simulink model "TST_EngPrt_PrtLimMech"  (R2016b)
settings: Solver=FixedStepDiscrete  StartTime=0.0  StopTime=simTime  FixedStep=sampleTime  RelTol=1e-3
values from neighbouring files (symbols this model uses):
  testCase = 1    [initTST_EngPrt_PrtLimMech_001.m]    (also in initTST_EngPrt_PrtLimMech_002.m = 2; initTST_EngPrt_PrtLimMech_003.m = 3; initTST_EngPrt_PrtLimMech_004.m = 4)
libraries: simulink x17, UnitTest_Lib x12
settings Model: Creator=zhengjinyan  LastModifiedBy=zhengjinyan
settings DebuggingCC: SignalRangeChecking=error

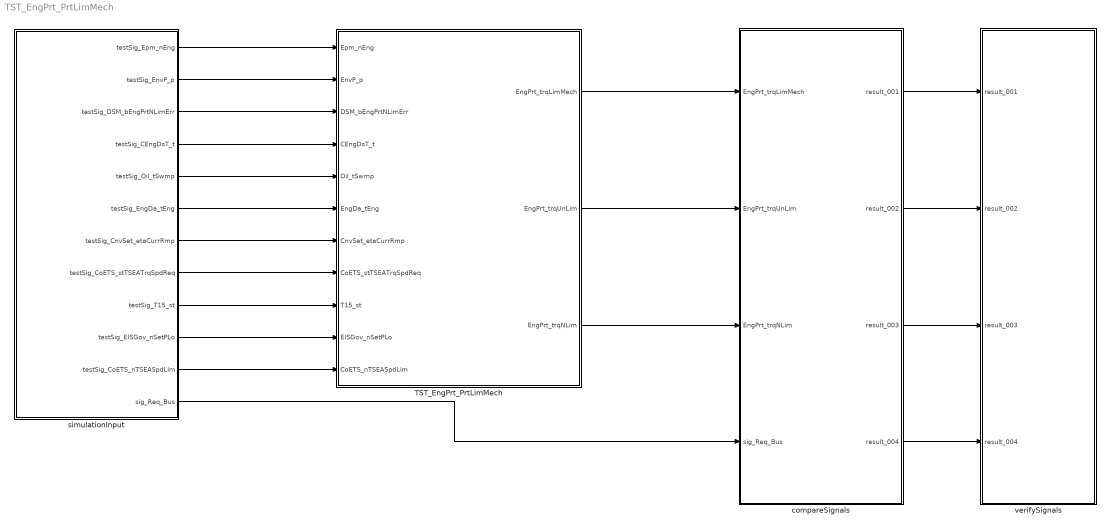
== system TST_EngPrt_PrtLimMech ==
  TST_EngPrt_PrtLimMech : Subsystem
  compareSignals : Subsystem
  simulationInput : Subsystem
  verifySignals : Subsystem
  wires:
  simulationInput/1(testSig_Epm_nEng) -> TST_EngPrt_PrtLimMech/1(Epm_nEng)
  simulationInput/2(testSig_EnvP_p) -> TST_EngPrt_PrtLimMech/2(EnvP_p)
  simulationInput/3(testSig_DSM_bEngPrtNLimErr) -> TST_EngPrt_PrtLimMech/3(DSM_bEngPrtNLimErr)
  simulationInput/4(testSig_CEngDsT_t) -> TST_EngPrt_PrtLimMech/4(CEngDsT_t)
  simulationInput/5(testSig_Oil_tSwmp) -> TST_EngPrt_PrtLimMech/5(Oil_tSwmp)
  simulationInput/6(testSig_EngDa_tEng) -> TST_EngPrt_PrtLimMech/6(EngDa_tEng)
  simulationInput/7(testSig_CnvSet_etaCurrRmp) -> TST_EngPrt_PrtLimMech/7(CnvSet_etaCurrRmp)
  simulationInput/8(testSig_CoETS_stTSEATrqSpdReq) -> TST_EngPrt_PrtLimMech/8(CoETS_stTSEATrqSpdReq)
  simulationInput/9(testSig_T15_st) -> TST_EngPrt_PrtLimMech/9(T15_st)
  simulationInput/10(testSig_EISGov_nSetPLo) -> TST_EngPrt_PrtLimMech/10(EISGov_nSetPLo)
  simulationInput/11(testSig_CoETS_nTSEASpdLim) -> TST_EngPrt_PrtLimMech/11(CoETS_nTSEASpdLim)
  TST_EngPrt_PrtLimMech/1(EngPrt_trqLimMech) -> compareSignals/1(EngPrt_trqLimMech)
  TST_EngPrt_PrtLimMech/2(EngPrt_trqUnLim) -> compareSignals/2(EngPrt_trqUnLim)
  TST_EngPrt_PrtLimMech/3(EngPrt_trqNLim) -> compareSignals/3(EngPrt_trqNLim)
  simulationInput/12(sig_Req_Bus) -> compareSignals/4(sig_Req_Bus)
  compareSignals/1(result_001) -> verifySignals/1(result_001)
  compareSignals/2(result_002) -> verifySignals/2(result_002)
  compareSignals/3(result_003) -> verifySignals/3(result_003)
  compareSignals/4(result_004) -> verifySignals/4(result_004)

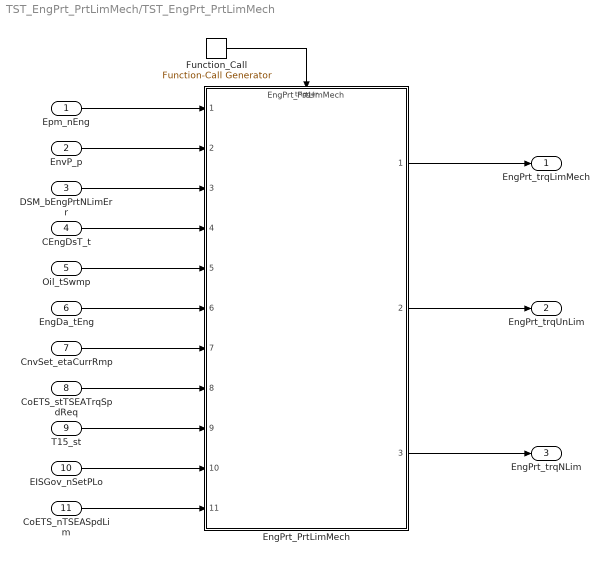
== system TST_EngPrt_PrtLimMech/TST_EngPrt_PrtLimMech ==
  Epm_nEng : Inport
  EnvP_p : Inport  Port=2
  DSM_bEngPrtNLimErr : Inport  Port=3
  CEngDsT_t : Inport  Port=4
  Oil_tSwmp : Inport  Port=5
  EngDa_tEng : Inport  Port=6
  CnvSet_etaCurrRmp : Inport  Port=7
  CoETS_stTSEATrqSpdReq : Inport  Port=8
  T15_st : Inport  Port=9
  EISGov_nSetPLo : Inport  Port=10
  CoETS_nTSEASpdLim : Inport  Port=11
  EngPrt_PrtLimMech : ModelReference  ModelNameDialog=EngPrt_PrtLimMech  SimulationMode=Normal  ModelReferenceVersion=1.43  TriggerPortName=function  TriggerPortTriggerType=function-call  TriggerPortStatesWhenEnabling=held
  Function_Call : simulink/Ports & Subsystems/Function-Call Generator  sample_time=sampleTime  numberOfIterations=1
  EngPrt_trqLimMech : Outport
  EngPrt_trqUnLim : Outport  Port=2
  EngPrt_trqNLim : Outport  Port=3
  wires:
  Function_Call/1 -> EngPrt_PrtLimMech/Trigger
  Epm_nEng/1 -> EngPrt_PrtLimMech/1
  EnvP_p/1 -> EngPrt_PrtLimMech/2
  DSM_bEngPrtNLimErr/1 -> EngPrt_PrtLimMech/3
  CEngDsT_t/1 -> EngPrt_PrtLimMech/4
  Oil_tSwmp/1 -> EngPrt_PrtLimMech/5
  EngDa_tEng/1 -> EngPrt_PrtLimMech/6
  CnvSet_etaCurrRmp/1 -> EngPrt_PrtLimMech/7
  CoETS_stTSEATrqSpdReq/1 -> EngPrt_PrtLimMech/8
  T15_st/1 -> EngPrt_PrtLimMech/9
  EISGov_nSetPLo/1 -> EngPrt_PrtLimMech/10
  CoETS_nTSEASpdLim/1 -> EngPrt_PrtLimMech/11
  EngPrt_PrtLimMech/1 -> EngPrt_trqLimMech/1
  EngPrt_PrtLimMech/2 -> EngPrt_trqUnLim/1
  EngPrt_PrtLimMech/3 -> EngPrt_trqNLim/1

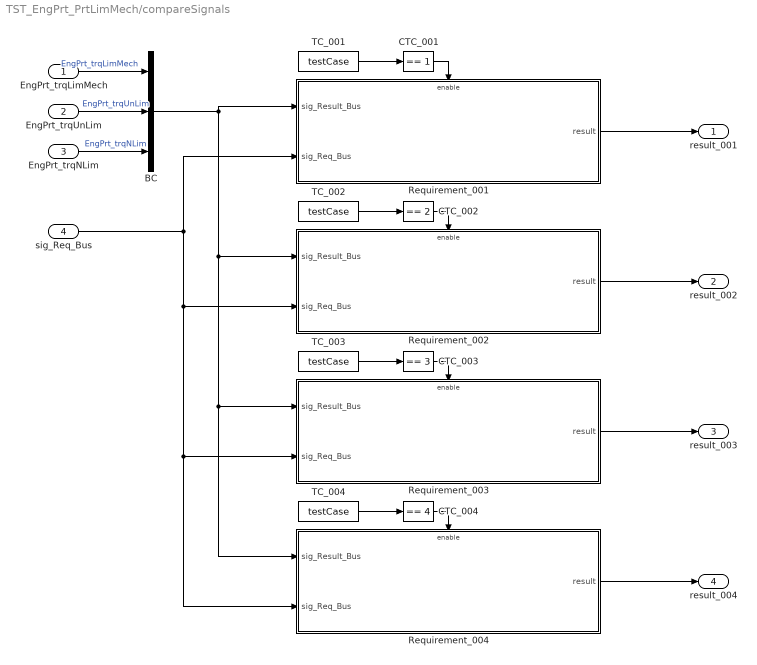
== system TST_EngPrt_PrtLimMech/compareSignals ==
  EngPrt_trqLimMech : Inport
  EngPrt_trqUnLim : Inport  Port=2
  EngPrt_trqNLim : Inport  Port=3
  sig_Req_Bus : Inport  Port=4
  BC : BusCreator  Inputs=3
  CTC_001 : simulink/Logic and Bit Operations/Compare To Constant  relop===  const=1  OutDataTypeStr=boolean
  CTC_002 : simulink/Logic and Bit Operations/Compare To Constant  relop===  const=2  OutDataTypeStr=boolean
  CTC_003 : simulink/Logic and Bit Operations/Compare To Constant  relop===  const=3  OutDataTypeStr=boolean
  CTC_004 : simulink/Logic and Bit Operations/Compare To Constant  relop===  const=4  OutDataTypeStr=boolean
  Requirement_001 : Subsystem
  Requirement_002 : Subsystem
  Requirement_003 : Subsystem
  Requirement_004 : Subsystem
  TC_001 : Constant  Value=testCase
  TC_002 : Constant  Value=testCase
  TC_003 : Constant  Value=testCase
  TC_004 : Constant  Value=testCase
  result_001 : Outport
  result_002 : Outport  Port=2
  result_003 : Outport  Port=3
  result_004 : Outport  Port=4
  wires:
  EngPrt_trqLimMech/1 -> BC/1  "EngPrt_trqLimMech"
  EngPrt_trqUnLim/1 -> BC/2  "EngPrt_trqUnLim"
  EngPrt_trqNLim/1 -> BC/3  "EngPrt_trqNLim"
  TC_001/1 -> CTC_001/1
  CTC_001/1 -> Requirement_001/Enable
  sig_Req_Bus/1 -> Requirement_003/2(sig_Req_Bus), Requirement_004/2(sig_Req_Bus), Requirement_002/2(sig_Req_Bus), Requirement_001/2(sig_Req_Bus)
  BC/1 -> Requirement_003/1(sig_Result_Bus), Requirement_004/1(sig_Result_Bus), Requirement_002/1(sig_Result_Bus), Requirement_001/1(sig_Result_Bus)
  Requirement_001/1(result) -> result_001/1
  TC_002/1 -> CTC_002/1
  CTC_002/1 -> Requirement_002/Enable
  Requirement_002/1(result) -> result_002/1
  TC_003/1 -> CTC_003/1
  CTC_003/1 -> Requirement_003/Enable
  Requirement_003/1(result) -> result_003/1
  TC_004/1 -> CTC_004/1
  CTC_004/1 -> Requirement_004/Enable
  Requirement_004/1(result) -> result_004/1

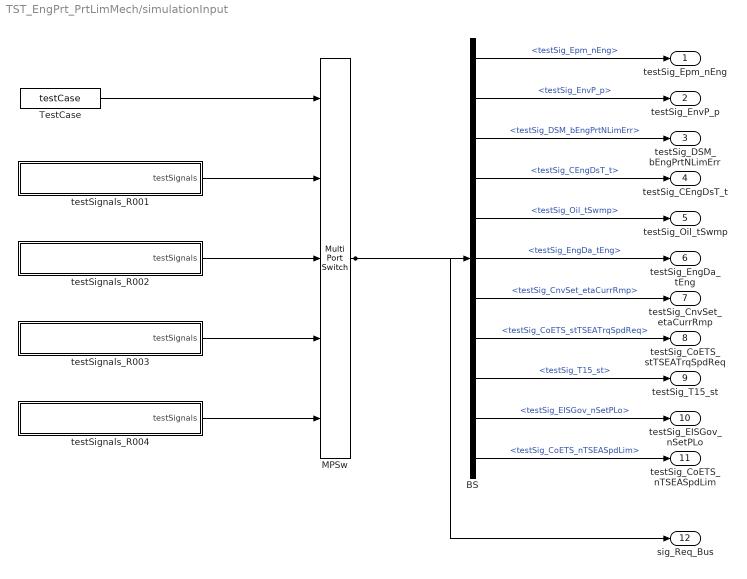
== system TST_EngPrt_PrtLimMech/simulationInput ==
  BS : BusSelector  OutputSignals=testSig_Epm_nEng,testSig_EnvP_p,testSig_DSM_bEngPrtNLimErr,testSig_CEngDsT_t,testSig_Oil_tSwmp,testSig_EngDa_tEng,testSig_CnvSet_etaCurrRmp,testSig_CoETS_stTSEATrqSpdReq,testSig_T15_st,testSig_EISGov_nSetPLo,testSig_CoETS_nTSEASpdLim
  MPSw : MultiPortSwitch  Inputs=4  SaturateOnIntegerOverflow=on  InputSameDT=on
  TestCase : Constant  Value=testCase
  testSignals_R001 : Subsystem
  testSignals_R002 : Subsystem
  testSignals_R003 : Subsystem
  testSignals_R004 : Subsystem
  testSig_Epm_nEng : Outport
  testSig_EnvP_p : Outport  Port=2
  testSig_DSM_bEngPrtNLimErr : Outport  Port=3
  testSig_CEngDsT_t : Outport  Port=4
  testSig_Oil_tSwmp : Outport  Port=5
  testSig_EngDa_tEng : Outport  Port=6
  testSig_CnvSet_etaCurrRmp : Outport  Port=7
  testSig_CoETS_stTSEATrqSpdReq : Outport  Port=8
  testSig_T15_st : Outport  Port=9
  testSig_EISGov_nSetPLo : Outport  Port=10
  testSig_CoETS_nTSEASpdLim : Outport  Port=11
  sig_Req_Bus : Outport  Port=12
  wires:
  BS/1 -> testSig_Epm_nEng/1  "<testSig_Epm_nEng>"
  BS/2 -> testSig_EnvP_p/1  "<testSig_EnvP_p>"
  BS/3 -> testSig_DSM_bEngPrtNLimErr/1  "<testSig_DSM_bEngPrtNLimErr>"
  BS/4 -> testSig_CEngDsT_t/1  "<testSig_CEngDsT_t>"
  BS/5 -> testSig_Oil_tSwmp/1  "<testSig_Oil_tSwmp>"
  BS/6 -> testSig_EngDa_tEng/1  "<testSig_EngDa_tEng>"
  BS/7 -> testSig_CnvSet_etaCurrRmp/1  "<testSig_CnvSet_etaCurrRmp>"
  BS/8 -> testSig_CoETS_stTSEATrqSpdReq/1  "<testSig_CoETS_stTSEATrqSpdReq>"
  BS/9 -> testSig_T15_st/1  "<testSig_T15_st>"
  BS/10 -> testSig_EISGov_nSetPLo/1  "<testSig_EISGov_nSetPLo>"
  BS/11 -> testSig_CoETS_nTSEASpdLim/1  "<testSig_CoETS_nTSEASpdLim>"
  MPSw/1 -> BS/1, sig_Req_Bus/1
  TestCase/1 -> MPSw/1
  testSignals_R001/1(testSignals) -> MPSw/2
  testSignals_R002/1(testSignals) -> MPSw/3
  testSignals_R003/1(testSignals) -> MPSw/4
  testSignals_R004/1(testSignals) -> MPSw/5

== system TST_EngPrt_PrtLimMech/verifySignals ==
  result_001 : Inport
  result_002 : Inport  Port=2
  result_003 : Inport  Port=3
  result_004 : Inport  Port=4
  Assertion_001 : Assertion  Enabled=off
  Assertion_002 : Assertion  Enabled=off
  Assertion_003 : Assertion  Enabled=off
  Assertion_004 : Assertion  Enabled=off
  wires:
  result_001/1 -> Assertion_001/1
  result_002/1 -> Assertion_002/1
  result_003/1 -> Assertion_003/1
  result_004/1 -> Assertion_004/1

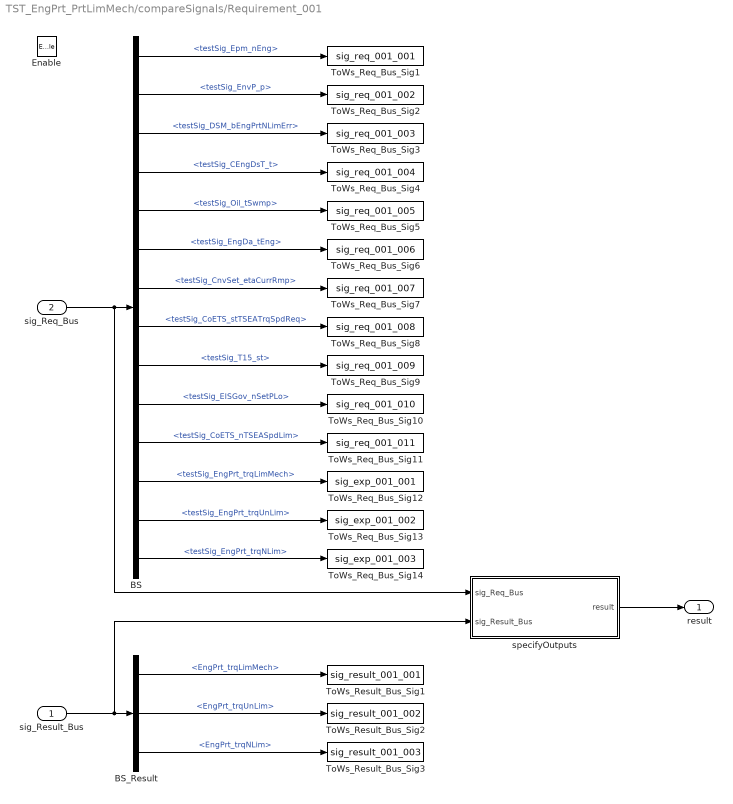
== system TST_EngPrt_PrtLimMech/compareSignals/Requirement_001 ==
  sig_Result_Bus : Inport
  sig_Req_Bus : Inport  Port=2
  Enable : EnablePort
  BS : BusSelector  OutputSignals=testSig_Epm_nEng,testSig_EnvP_p,testSig_DSM_bEngPrtNLimErr,testSig_CEngDsT_t,testSig_Oil_tSwmp,testSig_EngDa_tEng,testSig_CnvSet_etaCurrRmp,testSig_CoETS_stTSEATrqSpdReq,testSig_T15_st,testSig_EISGov_nSetPLo,testSig_CoETS_nTSEASpdLim,testSig_EngPrt_trqLimMech,testSig_EngPrt_trqUnLim,testSig_EngPrt_trqNLim
  BS_Result : BusSelector  OutputSignals=EngPrt_trqLimMech,EngPrt_trqUnLim,EngPrt_trqNLim
  ToWs_Req_Bus_Sig1 : ToWorkspace  VariableName=sig_req_001_001  SaveFormat=Structure With Time
  ToWs_Req_Bus_Sig10 : ToWorkspace  VariableName=sig_req_001_010  SaveFormat=Structure With Time
  ToWs_Req_Bus_Sig11 : ToWorkspace  VariableName=sig_req_001_011  SaveFormat=Structure With Time
  ToWs_Req_Bus_Sig12 : ToWorkspace  VariableName=sig_exp_001_001  SaveFormat=Structure With Time
  ToWs_Req_Bus_Sig13 : ToWorkspace  VariableName=sig_exp_001_002  SaveFormat=Structure With Time
  ToWs_Req_Bus_Sig14 : ToWorkspace  VariableName=sig_exp_001_003  SaveFormat=Structure With Time
  ToWs_Req_Bus_Sig2 : ToWorkspace  VariableName=sig_req_001_002  SaveFormat=Structure With Time
  ToWs_Req_Bus_Sig3 : ToWorkspace  VariableName=sig_req_001_003  SaveFormat=Structure With Time
  ToWs_Req_Bus_Sig4 : ToWorkspace  VariableName=sig_req_001_004  SaveFormat=Structure With Time
  ToWs_Req_Bus_Sig5 : ToWorkspace  VariableName=sig_req_001_005  SaveFormat=Structure With Time
  ToWs_Req_Bus_Sig6 : ToWorkspace  VariableName=sig_req_001_006  SaveFormat=Structure With Time
  ToWs_Req_Bus_Sig7 : ToWorkspace  VariableName=sig_req_001_007  SaveFormat=Structure With Time
  ToWs_Req_Bus_Sig8 : ToWorkspace  VariableName=sig_req_001_008  SaveFormat=Structure With Time
  ToWs_Req_Bus_Sig9 : ToWorkspace  VariableName=sig_req_001_009  SaveFormat=Structure With Time
  ToWs_Result_Bus_Sig1 : ToWorkspace  VariableName=sig_result_001_001  SaveFormat=Structure With Time
  ToWs_Result_Bus_Sig2 : ToWorkspace  VariableName=sig_result_001_002  SaveFormat=Structure With Time
  ToWs_Result_Bus_Sig3 : ToWorkspace  VariableName=sig_result_001_003  SaveFormat=Structure With Time
  specifyOutputs : Subsystem
  result : Outport
  wires:
  sig_Req_Bus/1 -> BS/1, specifyOutputs/1(sig_Req_Bus)
  BS/1 -> ToWs_Req_Bus_Sig1/1  "<testSig_Epm_nEng>"
  BS/2 -> ToWs_Req_Bus_Sig2/1  "<testSig_EnvP_p>"
  BS/3 -> ToWs_Req_Bus_Sig3/1  "<testSig_DSM_bEngPrtNLimErr>"
  BS/4 -> ToWs_Req_Bus_Sig4/1  "<testSig_CEngDsT_t>"
  BS/5 -> ToWs_Req_Bus_Sig5/1  "<testSig_Oil_tSwmp>"
  BS/6 -> ToWs_Req_Bus_Sig6/1  "<testSig_EngDa_tEng>"
  BS/7 -> ToWs_Req_Bus_Sig7/1  "<testSig_CnvSet_etaCurrRmp>"
  BS/8 -> ToWs_Req_Bus_Sig8/1  "<testSig_CoETS_stTSEATrqSpdReq>"
  BS/9 -> ToWs_Req_Bus_Sig9/1  "<testSig_T15_st>"
  BS/10 -> ToWs_Req_Bus_Sig10/1  "<testSig_EISGov_nSetPLo>"
  BS/11 -> ToWs_Req_Bus_Sig11/1  "<testSig_CoETS_nTSEASpdLim>"
  BS/12 -> ToWs_Req_Bus_Sig12/1  "<testSig_EngPrt_trqLimMech>"
  BS/13 -> ToWs_Req_Bus_Sig13/1  "<testSig_EngPrt_trqUnLim>"
  BS/14 -> ToWs_Req_Bus_Sig14/1  "<testSig_EngPrt_trqNLim>"
  sig_Result_Bus/1 -> BS_Result/1, specifyOutputs/2(sig_Result_Bus)
  BS_Result/1 -> ToWs_Result_Bus_Sig1/1  "<EngPrt_trqLimMech>"
  BS_Result/2 -> ToWs_Result_Bus_Sig2/1  "<EngPrt_trqUnLim>"
  BS_Result/3 -> ToWs_Result_Bus_Sig3/1  "<EngPrt_trqNLim>"
  specifyOutputs/1(result) -> result/1

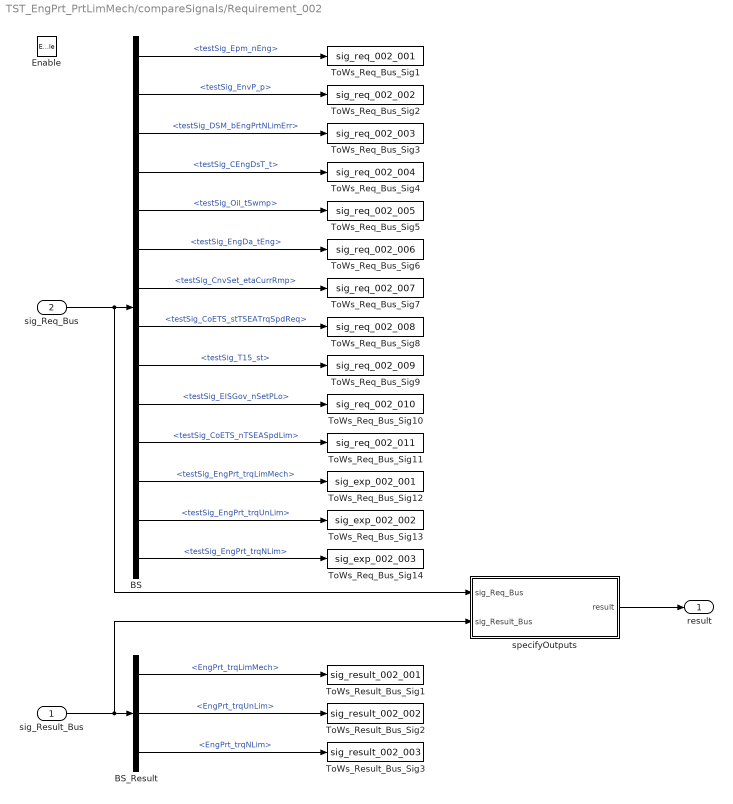
== system TST_EngPrt_PrtLimMech/compareSignals/Requirement_002 ==
  sig_Result_Bus : Inport
  sig_Req_Bus : Inport  Port=2
  Enable : EnablePort
  BS : BusSelector  OutputSignals=testSig_Epm_nEng,testSig_EnvP_p,testSig_DSM_bEngPrtNLimErr,testSig_CEngDsT_t,testSig_Oil_tSwmp,testSig_EngDa_tEng,testSig_CnvSet_etaCurrRmp,testSig_CoETS_stTSEATrqSpdReq,testSig_T15_st,testSig_EISGov_nSetPLo,testSig_CoETS_nTSEASpdLim,testSig_EngPrt_trqLimMech,testSig_EngPrt_trqUnLim,testSig_EngPrt_trqNLim
  BS_Result : BusSelector  OutputSignals=EngPrt_trqLimMech,EngPrt_trqUnLim,EngPrt_trqNLim
  ToWs_Req_Bus_Sig1 : ToWorkspace  VariableName=sig_req_002_001  SaveFormat=Structure With Time
  ToWs_Req_Bus_Sig10 : ToWorkspace  VariableName=sig_req_002_010  SaveFormat=Structure With Time
  ToWs_Req_Bus_Sig11 : ToWorkspace  VariableName=sig_req_002_011  SaveFormat=Structure With Time
  ToWs_Req_Bus_Sig12 : ToWorkspace  VariableName=sig_exp_002_001  SaveFormat=Structure With Time
  ToWs_Req_Bus_Sig13 : ToWorkspace  VariableName=sig_exp_002_002  SaveFormat=Structure With Time
  ToWs_Req_Bus_Sig14 : ToWorkspace  VariableName=sig_exp_002_003  SaveFormat=Structure With Time
  ToWs_Req_Bus_Sig2 : ToWorkspace  VariableName=sig_req_002_002  SaveFormat=Structure With Time
  ToWs_Req_Bus_Sig3 : ToWorkspace  VariableName=sig_req_002_003  SaveFormat=Structure With Time
  ToWs_Req_Bus_Sig4 : ToWorkspace  VariableName=sig_req_002_004  SaveFormat=Structure With Time
  ToWs_Req_Bus_Sig5 : ToWorkspace  VariableName=sig_req_002_005  SaveFormat=Structure With Time
  ToWs_Req_Bus_Sig6 : ToWorkspace  VariableName=sig_req_002_006  SaveFormat=Structure With Time
  ToWs_Req_Bus_Sig7 : ToWorkspace  VariableName=sig_req_002_007  SaveFormat=Structure With Time
  ToWs_Req_Bus_Sig8 : ToWorkspace  VariableName=sig_req_002_008  SaveFormat=Structure With Time
  ToWs_Req_Bus_Sig9 : ToWorkspace  VariableName=sig_req_002_009  SaveFormat=Structure With Time
  ToWs_Result_Bus_Sig1 : ToWorkspace  VariableName=sig_result_002_001  SaveFormat=Structure With Time
  ToWs_Result_Bus_Sig2 : ToWorkspace  VariableName=sig_result_002_002  SaveFormat=Structure With Time
  ToWs_Result_Bus_Sig3 : ToWorkspace  VariableName=sig_result_002_003  SaveFormat=Structure With Time
  specifyOutputs : Subsystem
  result : Outport
  wires:
  sig_Req_Bus/1 -> BS/1, specifyOutputs/1(sig_Req_Bus)
  BS/1 -> ToWs_Req_Bus_Sig1/1  "<testSig_Epm_nEng>"
  BS/2 -> ToWs_Req_Bus_Sig2/1  "<testSig_EnvP_p>"
  BS/3 -> ToWs_Req_Bus_Sig3/1  "<testSig_DSM_bEngPrtNLimErr>"
  BS/4 -> ToWs_Req_Bus_Sig4/1  "<testSig_CEngDsT_t>"
  BS/5 -> ToWs_Req_Bus_Sig5/1  "<testSig_Oil_tSwmp>"
  BS/6 -> ToWs_Req_Bus_Sig6/1  "<testSig_EngDa_tEng>"
  BS/7 -> ToWs_Req_Bus_Sig7/1  "<testSig_CnvSet_etaCurrRmp>"
  BS/8 -> ToWs_Req_Bus_Sig8/1  "<testSig_CoETS_stTSEATrqSpdReq>"
  BS/9 -> ToWs_Req_Bus_Sig9/1  "<testSig_T15_st>"
  BS/10 -> ToWs_Req_Bus_Sig10/1  "<testSig_EISGov_nSetPLo>"
  BS/11 -> ToWs_Req_Bus_Sig11/1  "<testSig_CoETS_nTSEASpdLim>"
  BS/12 -> ToWs_Req_Bus_Sig12/1  "<testSig_EngPrt_trqLimMech>"
  BS/13 -> ToWs_Req_Bus_Sig13/1  "<testSig_EngPrt_trqUnLim>"
  BS/14 -> ToWs_Req_Bus_Sig14/1  "<testSig_EngPrt_trqNLim>"
  sig_Result_Bus/1 -> BS_Result/1, specifyOutputs/2(sig_Result_Bus)
  BS_Result/1 -> ToWs_Result_Bus_Sig1/1  "<EngPrt_trqLimMech>"
  BS_Result/2 -> ToWs_Result_Bus_Sig2/1  "<EngPrt_trqUnLim>"
  BS_Result/3 -> ToWs_Result_Bus_Sig3/1  "<EngPrt_trqNLim>"
  specifyOutputs/1(result) -> result/1

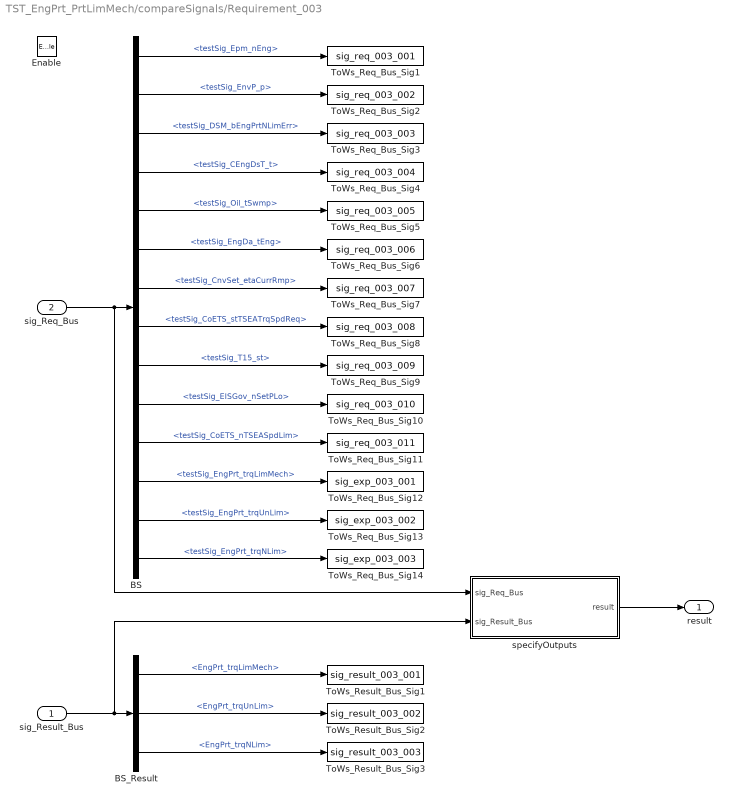
== system TST_EngPrt_PrtLimMech/compareSignals/Requirement_003 ==
  sig_Result_Bus : Inport
  sig_Req_Bus : Inport  Port=2
  Enable : EnablePort
  BS : BusSelector  OutputSignals=testSig_Epm_nEng,testSig_EnvP_p,testSig_DSM_bEngPrtNLimErr,testSig_CEngDsT_t,testSig_Oil_tSwmp,testSig_EngDa_tEng,testSig_CnvSet_etaCurrRmp,testSig_CoETS_stTSEATrqSpdReq,testSig_T15_st,testSig_EISGov_nSetPLo,testSig_CoETS_nTSEASpdLim,testSig_EngPrt_trqLimMech,testSig_EngPrt_trqUnLim,testSig_EngPrt_trqNLim
  BS_Result : BusSelector  OutputSignals=EngPrt_trqLimMech,EngPrt_trqUnLim,EngPrt_trqNLim
  ToWs_Req_Bus_Sig1 : ToWorkspace  VariableName=sig_req_003_001  SaveFormat=Structure With Time
  ToWs_Req_Bus_Sig10 : ToWorkspace  VariableName=sig_req_003_010  SaveFormat=Structure With Time
  ToWs_Req_Bus_Sig11 : ToWorkspace  VariableName=sig_req_003_011  SaveFormat=Structure With Time
  ToWs_Req_Bus_Sig12 : ToWorkspace  VariableName=sig_exp_003_001  SaveFormat=Structure With Time
  ToWs_Req_Bus_Sig13 : ToWorkspace  VariableName=sig_exp_003_002  SaveFormat=Structure With Time
  ToWs_Req_Bus_Sig14 : ToWorkspace  VariableName=sig_exp_003_003  SaveFormat=Structure With Time
  ToWs_Req_Bus_Sig2 : ToWorkspace  VariableName=sig_req_003_002  SaveFormat=Structure With Time
  ToWs_Req_Bus_Sig3 : ToWorkspace  VariableName=sig_req_003_003  SaveFormat=Structure With Time
  ToWs_Req_Bus_Sig4 : ToWorkspace  VariableName=sig_req_003_004  SaveFormat=Structure With Time
  ToWs_Req_Bus_Sig5 : ToWorkspace  VariableName=sig_req_003_005  SaveFormat=Structure With Time
  ToWs_Req_Bus_Sig6 : ToWorkspace  VariableName=sig_req_003_006  SaveFormat=Structure With Time
  ToWs_Req_Bus_Sig7 : ToWorkspace  VariableName=sig_req_003_007  SaveFormat=Structure With Time
  ToWs_Req_Bus_Sig8 : ToWorkspace  VariableName=sig_req_003_008  SaveFormat=Structure With Time
  ToWs_Req_Bus_Sig9 : ToWorkspace  VariableName=sig_req_003_009  SaveFormat=Structure With Time
  ToWs_Result_Bus_Sig1 : ToWorkspace  VariableName=sig_result_003_001  SaveFormat=Structure With Time
  ToWs_Result_Bus_Sig2 : ToWorkspace  VariableName=sig_result_003_002  SaveFormat=Structure With Time
  ToWs_Result_Bus_Sig3 : ToWorkspace  VariableName=sig_result_003_003  SaveFormat=Structure With Time
  specifyOutputs : Subsystem
  result : Outport
  wires:
  sig_Req_Bus/1 -> BS/1, specifyOutputs/1(sig_Req_Bus)
  BS/1 -> ToWs_Req_Bus_Sig1/1  "<testSig_Epm_nEng>"
  BS/2 -> ToWs_Req_Bus_Sig2/1  "<testSig_EnvP_p>"
  BS/3 -> ToWs_Req_Bus_Sig3/1  "<testSig_DSM_bEngPrtNLimErr>"
  BS/4 -> ToWs_Req_Bus_Sig4/1  "<testSig_CEngDsT_t>"
  BS/5 -> ToWs_Req_Bus_Sig5/1  "<testSig_Oil_tSwmp>"
  BS/6 -> ToWs_Req_Bus_Sig6/1  "<testSig_EngDa_tEng>"
  BS/7 -> ToWs_Req_Bus_Sig7/1  "<testSig_CnvSet_etaCurrRmp>"
  BS/8 -> ToWs_Req_Bus_Sig8/1  "<testSig_CoETS_stTSEATrqSpdReq>"
  BS/9 -> ToWs_Req_Bus_Sig9/1  "<testSig_T15_st>"
  BS/10 -> ToWs_Req_Bus_Sig10/1  "<testSig_EISGov_nSetPLo>"
  BS/11 -> ToWs_Req_Bus_Sig11/1  "<testSig_CoETS_nTSEASpdLim>"
  BS/12 -> ToWs_Req_Bus_Sig12/1  "<testSig_EngPrt_trqLimMech>"
  BS/13 -> ToWs_Req_Bus_Sig13/1  "<testSig_EngPrt_trqUnLim>"
  BS/14 -> ToWs_Req_Bus_Sig14/1  "<testSig_EngPrt_trqNLim>"
  sig_Result_Bus/1 -> BS_Result/1, specifyOutputs/2(sig_Result_Bus)
  BS_Result/1 -> ToWs_Result_Bus_Sig1/1  "<EngPrt_trqLimMech>"
  BS_Result/2 -> ToWs_Result_Bus_Sig2/1  "<EngPrt_trqUnLim>"
  BS_Result/3 -> ToWs_Result_Bus_Sig3/1  "<EngPrt_trqNLim>"
  specifyOutputs/1(result) -> result/1

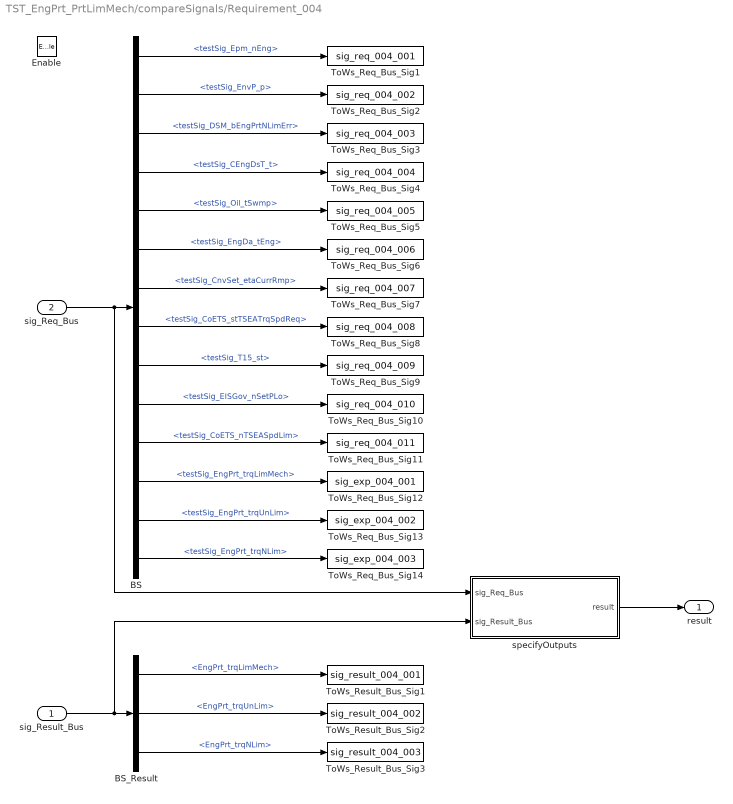
== system TST_EngPrt_PrtLimMech/compareSignals/Requirement_004 ==
  sig_Result_Bus : Inport
  sig_Req_Bus : Inport  Port=2
  Enable : EnablePort
  BS : BusSelector  OutputSignals=testSig_Epm_nEng,testSig_EnvP_p,testSig_DSM_bEngPrtNLimErr,testSig_CEngDsT_t,testSig_Oil_tSwmp,testSig_EngDa_tEng,testSig_CnvSet_etaCurrRmp,testSig_CoETS_stTSEATrqSpdReq,testSig_T15_st,testSig_EISGov_nSetPLo,testSig_CoETS_nTSEASpdLim,testSig_EngPrt_trqLimMech,testSig_EngPrt_trqUnLim,testSig_EngPrt_trqNLim
  BS_Result : BusSelector  OutputSignals=EngPrt_trqLimMech,EngPrt_trqUnLim,EngPrt_trqNLim
  ToWs_Req_Bus_Sig1 : ToWorkspace  VariableName=sig_req_004_001  SaveFormat=Structure With Time
  ToWs_Req_Bus_Sig10 : ToWorkspace  VariableName=sig_req_004_010  SaveFormat=Structure With Time
  ToWs_Req_Bus_Sig11 : ToWorkspace  VariableName=sig_req_004_011  SaveFormat=Structure With Time
  ToWs_Req_Bus_Sig12 : ToWorkspace  VariableName=sig_exp_004_001  SaveFormat=Structure With Time
  ToWs_Req_Bus_Sig13 : ToWorkspace  VariableName=sig_exp_004_002  SaveFormat=Structure With Time
  ToWs_Req_Bus_Sig14 : ToWorkspace  VariableName=sig_exp_004_003  SaveFormat=Structure With Time
  ToWs_Req_Bus_Sig2 : ToWorkspace  VariableName=sig_req_004_002  SaveFormat=Structure With Time
  ToWs_Req_Bus_Sig3 : ToWorkspace  VariableName=sig_req_004_003  SaveFormat=Structure With Time
  ToWs_Req_Bus_Sig4 : ToWorkspace  VariableName=sig_req_004_004  SaveFormat=Structure With Time
  ToWs_Req_Bus_Sig5 : ToWorkspace  VariableName=sig_req_004_005  SaveFormat=Structure With Time
  ToWs_Req_Bus_Sig6 : ToWorkspace  VariableName=sig_req_004_006  SaveFormat=Structure With Time
  ToWs_Req_Bus_Sig7 : ToWorkspace  VariableName=sig_req_004_007  SaveFormat=Structure With Time
  ToWs_Req_Bus_Sig8 : ToWorkspace  VariableName=sig_req_004_008  SaveFormat=Structure With Time
  ToWs_Req_Bus_Sig9 : ToWorkspace  VariableName=sig_req_004_009  SaveFormat=Structure With Time
  ToWs_Result_Bus_Sig1 : ToWorkspace  VariableName=sig_result_004_001  SaveFormat=Structure With Time
  ToWs_Result_Bus_Sig2 : ToWorkspace  VariableName=sig_result_004_002  SaveFormat=Structure With Time
  ToWs_Result_Bus_Sig3 : ToWorkspace  VariableName=sig_result_004_003  SaveFormat=Structure With Time
  specifyOutputs : Subsystem
  result : Outport
  wires:
  sig_Req_Bus/1 -> BS/1, specifyOutputs/1(sig_Req_Bus)
  BS/1 -> ToWs_Req_Bus_Sig1/1  "<testSig_Epm_nEng>"
  BS/2 -> ToWs_Req_Bus_Sig2/1  "<testSig_EnvP_p>"
  BS/3 -> ToWs_Req_Bus_Sig3/1  "<testSig_DSM_bEngPrtNLimErr>"
  BS/4 -> ToWs_Req_Bus_Sig4/1  "<testSig_CEngDsT_t>"
  BS/5 -> ToWs_Req_Bus_Sig5/1  "<testSig_Oil_tSwmp>"
  BS/6 -> ToWs_Req_Bus_Sig6/1  "<testSig_EngDa_tEng>"
  BS/7 -> ToWs_Req_Bus_Sig7/1  "<testSig_CnvSet_etaCurrRmp>"
  BS/8 -> ToWs_Req_Bus_Sig8/1  "<testSig_CoETS_stTSEATrqSpdReq>"
  BS/9 -> ToWs_Req_Bus_Sig9/1  "<testSig_T15_st>"
  BS/10 -> ToWs_Req_Bus_Sig10/1  "<testSig_EISGov_nSetPLo>"
  BS/11 -> ToWs_Req_Bus_Sig11/1  "<testSig_CoETS_nTSEASpdLim>"
  BS/12 -> ToWs_Req_Bus_Sig12/1  "<testSig_EngPrt_trqLimMech>"
  BS/13 -> ToWs_Req_Bus_Sig13/1  "<testSig_EngPrt_trqUnLim>"
  BS/14 -> ToWs_Req_Bus_Sig14/1  "<testSig_EngPrt_trqNLim>"
  sig_Result_Bus/1 -> BS_Result/1, specifyOutputs/2(sig_Result_Bus)
  BS_Result/1 -> ToWs_Result_Bus_Sig1/1  "<EngPrt_trqLimMech>"
  BS_Result/2 -> ToWs_Result_Bus_Sig2/1  "<EngPrt_trqUnLim>"
  BS_Result/3 -> ToWs_Result_Bus_Sig3/1  "<EngPrt_trqNLim>"
  specifyOutputs/1(result) -> result/1

== system TST_EngPrt_PrtLimMech/simulationInput/testSignals_R001 ==
  BC : BusCreator  Inputs=14
  spec_CEngDsT_t : FromWorkspace  VariableName=testSig_CEngDsT_t  Interpolate=off  OutputAfterFinalValue=Holding final value
  spec_CnvSet_etaCurrRmp : FromWorkspace  VariableName=testSig_CnvSet_etaCurrRmp  Interpolate=off  OutputAfterFinalValue=Holding final value
  spec_CoETS_nTSEASpdLim : FromWorkspace  VariableName=testSig_CoETS_nTSEASpdLim  Interpolate=off  OutputAfterFinalValue=Holding final value
  spec_CoETS_stTSEATrqSpdReq : FromWorkspace  VariableName=testSig_CoETS_stTSEATrqSpdReq  Interpolate=off  OutputAfterFinalValue=Holding final value
  spec_DSM_bEngPrtNLimErr : FromWorkspace  VariableName=testSig_DSM_bEngPrtNLimErr  Interpolate=off  OutputAfterFinalValue=Holding final value
  spec_EISGov_nSetPLo : FromWorkspace  VariableName=testSig_EISGov_nSetPLo  Interpolate=off  OutputAfterFinalValue=Holding final value
  spec_EngDa_tEng : FromWorkspace  VariableName=testSig_EngDa_tEng  Interpolate=off  OutputAfterFinalValue=Holding final value
  spec_EngPrt_trqLimMech : FromWorkspace  VariableName=testSig_EngPrt_trqLimMech  Interpolate=off  OutputAfterFinalValue=Holding final value
  spec_EngPrt_trqNLim : FromWorkspace  VariableName=testSig_EngPrt_trqNLim  Interpolate=off  OutputAfterFinalValue=Holding final value
  spec_EngPrt_trqUnLim : FromWorkspace  VariableName=testSig_EngPrt_trqUnLim  Interpolate=off  OutputAfterFinalValue=Holding final value
  spec_EnvP_p : FromWorkspace  VariableName=testSig_EnvP_p  Interpolate=off  OutputAfterFinalValue=Holding final value
  spec_Epm_nEng : FromWorkspace  VariableName=testSig_Epm_nEng  Interpolate=off  OutputAfterFinalValue=Holding final value
  spec_Oil_tSwmp : FromWorkspace  VariableName=testSig_Oil_tSwmp  Interpolate=off  OutputAfterFinalValue=Holding final value
  spec_T15_st : FromWorkspace  VariableName=testSig_T15_st  Interpolate=off  OutputAfterFinalValue=Holding final value
  testSignals : Outport
  wires:
  BC/1 -> testSignals/1
  spec_Epm_nEng/1 -> BC/1  "testSig_Epm_nEng"
  spec_EnvP_p/1 -> BC/2  "testSig_EnvP_p"
  spec_DSM_bEngPrtNLimErr/1 -> BC/3  "testSig_DSM_bEngPrtNLimErr"
  spec_CEngDsT_t/1 -> BC/4  "testSig_CEngDsT_t"
  spec_Oil_tSwmp/1 -> BC/5  "testSig_Oil_tSwmp"
  spec_EngDa_tEng/1 -> BC/6  "testSig_EngDa_tEng"
  spec_CnvSet_etaCurrRmp/1 -> BC/7  "testSig_CnvSet_etaCurrRmp"
  spec_CoETS_stTSEATrqSpdReq/1 -> BC/8  "testSig_CoETS_stTSEATrqSpdReq"
  spec_T15_st/1 -> BC/9  "testSig_T15_st"
  spec_EISGov_nSetPLo/1 -> BC/10  "testSig_EISGov_nSetPLo"
  spec_CoETS_nTSEASpdLim/1 -> BC/11  "testSig_CoETS_nTSEASpdLim"
  spec_EngPrt_trqLimMech/1 -> BC/12  "testSig_EngPrt_trqLimMech"
  spec_EngPrt_trqUnLim/1 -> BC/13  "testSig_EngPrt_trqUnLim"
  spec_EngPrt_trqNLim/1 -> BC/14  "testSig_EngPrt_trqNLim"

== system TST_EngPrt_PrtLimMech/simulationInput/testSignals_R002 ==
  BC : BusCreator  Inputs=14
  spec_CEngDsT_t : FromWorkspace  VariableName=testSig_CEngDsT_t  Interpolate=off  OutputAfterFinalValue=Holding final value
  spec_CnvSet_etaCurrRmp : FromWorkspace  VariableName=testSig_CnvSet_etaCurrRmp  Interpolate=off  OutputAfterFinalValue=Holding final value
  spec_CoETS_nTSEASpdLim : FromWorkspace  VariableName=testSig_CoETS_nTSEASpdLim  Interpolate=off  OutputAfterFinalValue=Holding final value
  spec_CoETS_stTSEATrqSpdReq : FromWorkspace  VariableName=testSig_CoETS_stTSEATrqSpdReq  Interpolate=off  OutputAfterFinalValue=Holding final value
  spec_DSM_bEngPrtNLimErr : FromWorkspace  VariableName=testSig_DSM_bEngPrtNLimErr  Interpolate=off  OutputAfterFinalValue=Holding final value
  spec_EISGov_nSetPLo : FromWorkspace  VariableName=testSig_EISGov_nSetPLo  Interpolate=off  OutputAfterFinalValue=Holding final value
  spec_EngDa_tEng : FromWorkspace  VariableName=testSig_EngDa_tEng  Interpolate=off  OutputAfterFinalValue=Holding final value
  spec_EngPrt_trqLimMech : FromWorkspace  VariableName=testSig_EngPrt_trqLimMech  Interpolate=off  OutputAfterFinalValue=Holding final value
  spec_EngPrt_trqNLim : FromWorkspace  VariableName=testSig_EngPrt_trqNLim  Interpolate=off  OutputAfterFinalValue=Holding final value
  spec_EngPrt_trqUnLim : FromWorkspace  VariableName=testSig_EngPrt_trqUnLim  Interpolate=off  OutputAfterFinalValue=Holding final value
  spec_EnvP_p : FromWorkspace  VariableName=testSig_EnvP_p  Interpolate=off  OutputAfterFinalValue=Holding final value
  spec_Epm_nEng : FromWorkspace  VariableName=testSig_Epm_nEng  Interpolate=off  OutputAfterFinalValue=Holding final value
  spec_Oil_tSwmp : FromWorkspace  VariableName=testSig_Oil_tSwmp  Interpolate=off  OutputAfterFinalValue=Holding final value
  spec_T15_st : FromWorkspace  VariableName=testSig_T15_st  Interpolate=off  OutputAfterFinalValue=Holding final value
  testSignals : Outport
  wires:
  BC/1 -> testSignals/1
  spec_Epm_nEng/1 -> BC/1  "testSig_Epm_nEng"
  spec_EnvP_p/1 -> BC/2  "testSig_EnvP_p"
  spec_DSM_bEngPrtNLimErr/1 -> BC/3  "testSig_DSM_bEngPrtNLimErr"
  spec_CEngDsT_t/1 -> BC/4  "testSig_CEngDsT_t"
  spec_Oil_tSwmp/1 -> BC/5  "testSig_Oil_tSwmp"
  spec_EngDa_tEng/1 -> BC/6  "testSig_EngDa_tEng"
  spec_CnvSet_etaCurrRmp/1 -> BC/7  "testSig_CnvSet_etaCurrRmp"
  spec_CoETS_stTSEATrqSpdReq/1 -> BC/8  "testSig_CoETS_stTSEATrqSpdReq"
  spec_T15_st/1 -> BC/9  "testSig_T15_st"
  spec_EISGov_nSetPLo/1 -> BC/10  "testSig_EISGov_nSetPLo"
  spec_CoETS_nTSEASpdLim/1 -> BC/11  "testSig_CoETS_nTSEASpdLim"
  spec_EngPrt_trqLimMech/1 -> BC/12  "testSig_EngPrt_trqLimMech"
  spec_EngPrt_trqUnLim/1 -> BC/13  "testSig_EngPrt_trqUnLim"
  spec_EngPrt_trqNLim/1 -> BC/14  "testSig_EngPrt_trqNLim"

== system TST_EngPrt_PrtLimMech/simulationInput/testSignals_R003 ==
  BC : BusCreator  Inputs=14
  spec_CEngDsT_t : FromWorkspace  VariableName=testSig_CEngDsT_t  Interpolate=off  OutputAfterFinalValue=Holding final value
  spec_CnvSet_etaCurrRmp : FromWorkspace  VariableName=testSig_CnvSet_etaCurrRmp  Interpolate=off  OutputAfterFinalValue=Holding final value
  spec_CoETS_nTSEASpdLim : FromWorkspace  VariableName=testSig_CoETS_nTSEASpdLim  Interpolate=off  OutputAfterFinalValue=Holding final value
  spec_CoETS_stTSEATrqSpdReq : FromWorkspace  VariableName=testSig_CoETS_stTSEATrqSpdReq  Interpolate=off  OutputAfterFinalValue=Holding final value
  spec_DSM_bEngPrtNLimErr : FromWorkspace  VariableName=testSig_DSM_bEngPrtNLimErr  Interpolate=off  OutputAfterFinalValue=Holding final value
  spec_EISGov_nSetPLo : FromWorkspace  VariableName=testSig_EISGov_nSetPLo  Interpolate=off  OutputAfterFinalValue=Holding final value
  spec_EngDa_tEng : FromWorkspace  VariableName=testSig_EngDa_tEng  Interpolate=off  OutputAfterFinalValue=Holding final value
  spec_EngPrt_trqLimMech : FromWorkspace  VariableName=testSig_EngPrt_trqLimMech  Interpolate=off  OutputAfterFinalValue=Holding final value
  spec_EngPrt_trqNLim : FromWorkspace  VariableName=testSig_EngPrt_trqNLim  Interpolate=off  OutputAfterFinalValue=Holding final value
  spec_EngPrt_trqUnLim : FromWorkspace  VariableName=testSig_EngPrt_trqUnLim  Interpolate=off  OutputAfterFinalValue=Holding final value
  spec_EnvP_p : FromWorkspace  VariableName=testSig_EnvP_p  Interpolate=off  OutputAfterFinalValue=Holding final value
  spec_Epm_nEng : FromWorkspace  VariableName=testSig_Epm_nEng  Interpolate=off  OutputAfterFinalValue=Holding final value
  spec_Oil_tSwmp : FromWorkspace  VariableName=testSig_Oil_tSwmp  Interpolate=off  OutputAfterFinalValue=Holding final value
  spec_T15_st : FromWorkspace  VariableName=testSig_T15_st  Interpolate=off  OutputAfterFinalValue=Holding final value
  testSignals : Outport
  wires:
  BC/1 -> testSignals/1
  spec_Epm_nEng/1 -> BC/1  "testSig_Epm_nEng"
  spec_EnvP_p/1 -> BC/2  "testSig_EnvP_p"
  spec_DSM_bEngPrtNLimErr/1 -> BC/3  "testSig_DSM_bEngPrtNLimErr"
  spec_CEngDsT_t/1 -> BC/4  "testSig_CEngDsT_t"
  spec_Oil_tSwmp/1 -> BC/5  "testSig_Oil_tSwmp"
  spec_EngDa_tEng/1 -> BC/6  "testSig_EngDa_tEng"
  spec_CnvSet_etaCurrRmp/1 -> BC/7  "testSig_CnvSet_etaCurrRmp"
  spec_CoETS_stTSEATrqSpdReq/1 -> BC/8  "testSig_CoETS_stTSEATrqSpdReq"
  spec_T15_st/1 -> BC/9  "testSig_T15_st"
  spec_EISGov_nSetPLo/1 -> BC/10  "testSig_EISGov_nSetPLo"
  spec_CoETS_nTSEASpdLim/1 -> BC/11  "testSig_CoETS_nTSEASpdLim"
  spec_EngPrt_trqLimMech/1 -> BC/12  "testSig_EngPrt_trqLimMech"
  spec_EngPrt_trqUnLim/1 -> BC/13  "testSig_EngPrt_trqUnLim"
  spec_EngPrt_trqNLim/1 -> BC/14  "testSig_EngPrt_trqNLim"

== system TST_EngPrt_PrtLimMech/simulationInput/testSignals_R004 ==
  BC : BusCreator  Inputs=14
  spec_CEngDsT_t : FromWorkspace  VariableName=testSig_CEngDsT_t  Interpolate=off  OutputAfterFinalValue=Holding final value
  spec_CnvSet_etaCurrRmp : FromWorkspace  VariableName=testSig_CnvSet_etaCurrRmp  Interpolate=off  OutputAfterFinalValue=Holding final value
  spec_CoETS_nTSEASpdLim : FromWorkspace  VariableName=testSig_CoETS_nTSEASpdLim  Interpolate=off  OutputAfterFinalValue=Holding final value
  spec_CoETS_stTSEATrqSpdReq : FromWorkspace  VariableName=testSig_CoETS_stTSEATrqSpdReq  Interpolate=off  OutputAfterFinalValue=Holding final value
  spec_DSM_bEngPrtNLimErr : FromWorkspace  VariableName=testSig_DSM_bEngPrtNLimErr  Interpolate=off  OutputAfterFinalValue=Holding final value
  spec_EISGov_nSetPLo : FromWorkspace  VariableName=testSig_EISGov_nSetPLo  Interpolate=off  OutputAfterFinalValue=Holding final value
  spec_EngDa_tEng : FromWorkspace  VariableName=testSig_EngDa_tEng  Interpolate=off  OutputAfterFinalValue=Holding final value
  spec_EngPrt_trqLimMech : FromWorkspace  VariableName=testSig_EngPrt_trqLimMech  Interpolate=off  OutputAfterFinalValue=Holding final value
  spec_EngPrt_trqNLim : FromWorkspace  VariableName=testSig_EngPrt_trqNLim  Interpolate=off  OutputAfterFinalValue=Holding final value
  spec_EngPrt_trqUnLim : FromWorkspace  VariableName=testSig_EngPrt_trqUnLim  Interpolate=off  OutputAfterFinalValue=Holding final value
  spec_EnvP_p : FromWorkspace  VariableName=testSig_EnvP_p  Interpolate=off  OutputAfterFinalValue=Holding final value
  spec_Epm_nEng : FromWorkspace  VariableName=testSig_Epm_nEng  Interpolate=off  OutputAfterFinalValue=Holding final value
  spec_Oil_tSwmp : FromWorkspace  VariableName=testSig_Oil_tSwmp  Interpolate=off  OutputAfterFinalValue=Holding final value
  spec_T15_st : FromWorkspace  VariableName=testSig_T15_st  Interpolate=off  OutputAfterFinalValue=Holding final value
  testSignals : Outport
  wires:
  BC/1 -> testSignals/1
  spec_Epm_nEng/1 -> BC/1  "testSig_Epm_nEng"
  spec_EnvP_p/1 -> BC/2  "testSig_EnvP_p"
  spec_DSM_bEngPrtNLimErr/1 -> BC/3  "testSig_DSM_bEngPrtNLimErr"
  spec_CEngDsT_t/1 -> BC/4  "testSig_CEngDsT_t"
  spec_Oil_tSwmp/1 -> BC/5  "testSig_Oil_tSwmp"
  spec_EngDa_tEng/1 -> BC/6  "testSig_EngDa_tEng"
  spec_CnvSet_etaCurrRmp/1 -> BC/7  "testSig_CnvSet_etaCurrRmp"
  spec_CoETS_stTSEATrqSpdReq/1 -> BC/8  "testSig_CoETS_stTSEATrqSpdReq"
  spec_T15_st/1 -> BC/9  "testSig_T15_st"
  spec_EISGov_nSetPLo/1 -> BC/10  "testSig_EISGov_nSetPLo"
  spec_CoETS_nTSEASpdLim/1 -> BC/11  "testSig_CoETS_nTSEASpdLim"
  spec_EngPrt_trqLimMech/1 -> BC/12  "testSig_EngPrt_trqLimMech"
  spec_EngPrt_trqUnLim/1 -> BC/13  "testSig_EngPrt_trqUnLim"
  spec_EngPrt_trqNLim/1 -> BC/14  "testSig_EngPrt_trqNLim"

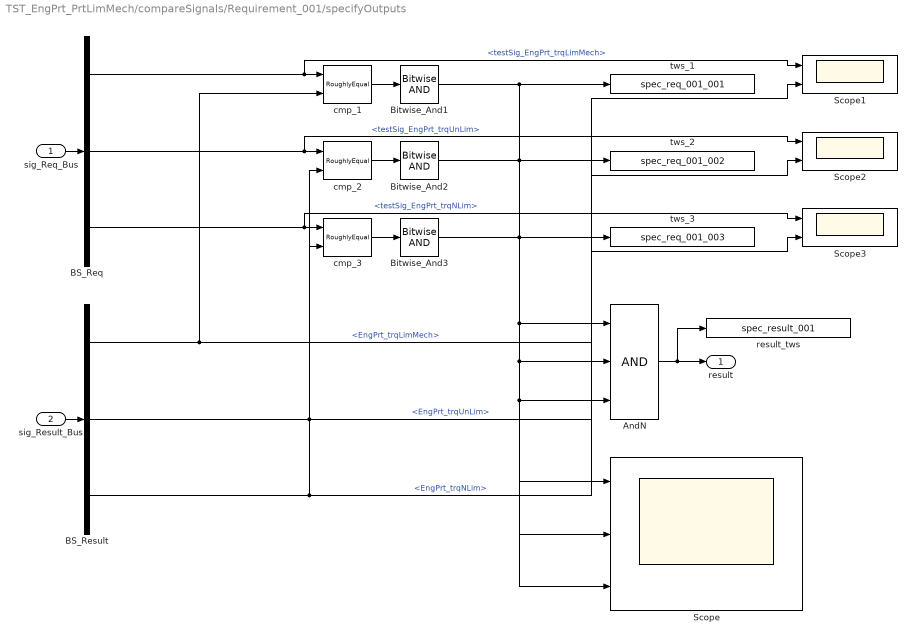
== system TST_EngPrt_PrtLimMech/compareSignals/Requirement_001/specifyOutputs ==
  sig_Req_Bus : Inport
  sig_Result_Bus : Inport  Port=2
  AndN : Logic  Inputs=3
  BS_Req : BusSelector  OutputSignals=testSig_EngPrt_trqLimMech,testSig_EngPrt_trqUnLim,testSig_EngPrt_trqNLim
  BS_Result : BusSelector  OutputSignals=EngPrt_trqLimMech,EngPrt_trqUnLim,EngPrt_trqNLim
  Bitwise_And1 : simulink/Logic and Bit Operations/Bitwise Operator  logicop=AND  UseBitMask=off  BitMask=bin2dec('11011001')  BitMaskRealWorld=Stored Integer
  Bitwise_And2 : simulink/Logic and Bit Operations/Bitwise Operator  logicop=AND  UseBitMask=off  BitMask=bin2dec('11011001')  BitMaskRealWorld=Stored Integer
  Bitwise_And3 : simulink/Logic and Bit Operations/Bitwise Operator  logicop=AND  UseBitMask=off  BitMask=bin2dec('11011001')  BitMaskRealWorld=Stored Integer
  Scope : Scope  NumInputPorts=3
  Scope1 : Scope  NumInputPorts=2
  Scope2 : Scope  NumInputPorts=2
  Scope3 : Scope  NumInputPorts=2
  cmp_1 : UnitTest_Lib/RoughlyEqual  slope=1
  cmp_2 : UnitTest_Lib/RoughlyEqual  slope=0.1
  cmp_3 : UnitTest_Lib/RoughlyEqual  slope=1
  result_tws : ToWorkspace  VariableName=spec_result_001
  tws_1 : ToWorkspace  VariableName=spec_req_001_001
  tws_2 : ToWorkspace  VariableName=spec_req_001_002
  tws_3 : ToWorkspace  VariableName=spec_req_001_003
  result : Outport
  wires:
  sig_Req_Bus/1 -> BS_Req/1
  sig_Result_Bus/1 -> BS_Result/1
  AndN/1 -> result/1, result_tws/1
  BS_Req/1 -> cmp_1/1, Scope1/1  "<testSig_EngPrt_trqLimMech>"
  BS_Result/1 -> cmp_1/2, Scope1/2  "<EngPrt_trqLimMech>"
  cmp_1/1 -> Bitwise_And1/1
  Bitwise_And1/1 -> AndN/1, Scope/1, tws_1/1
  BS_Req/2 -> cmp_2/1, Scope2/1  "<testSig_EngPrt_trqUnLim>"
  BS_Result/2 -> cmp_2/2, Scope2/2  "<EngPrt_trqUnLim>"
  cmp_2/1 -> Bitwise_And2/1
  Bitwise_And2/1 -> AndN/2, Scope/2, tws_2/1
  BS_Req/3 -> cmp_3/1, Scope3/1  "<testSig_EngPrt_trqNLim>"
  BS_Result/3 -> cmp_3/2, Scope3/2  "<EngPrt_trqNLim>"
  cmp_3/1 -> Bitwise_And3/1
  Bitwise_And3/1 -> AndN/3, Scope/3, tws_3/1

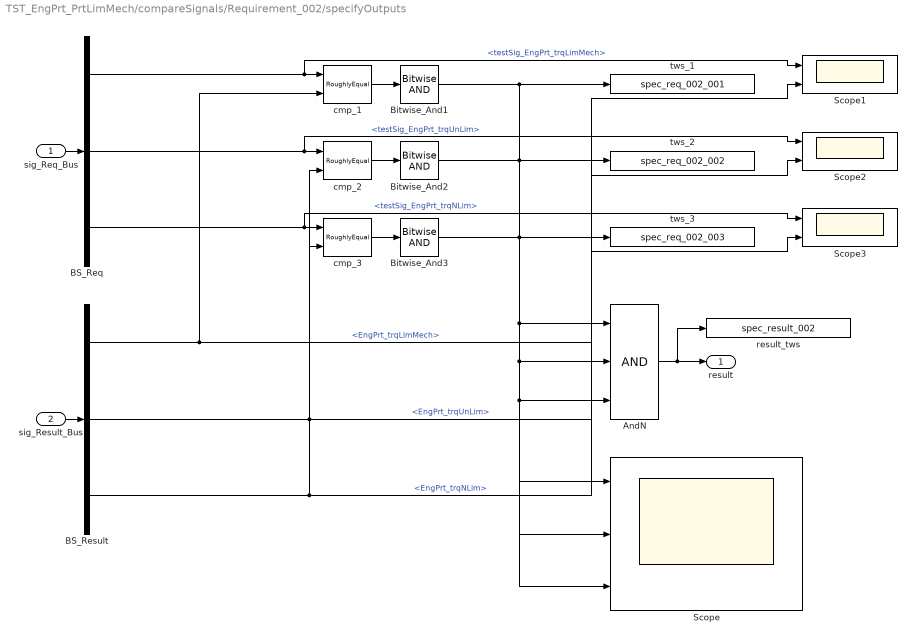
== system TST_EngPrt_PrtLimMech/compareSignals/Requirement_002/specifyOutputs ==
  sig_Req_Bus : Inport
  sig_Result_Bus : Inport  Port=2
  AndN : Logic  Inputs=3
  BS_Req : BusSelector  OutputSignals=testSig_EngPrt_trqLimMech,testSig_EngPrt_trqUnLim,testSig_EngPrt_trqNLim
  BS_Result : BusSelector  OutputSignals=EngPrt_trqLimMech,EngPrt_trqUnLim,EngPrt_trqNLim
  Bitwise_And1 : simulink/Logic and Bit Operations/Bitwise Operator  logicop=AND  UseBitMask=off  BitMask=bin2dec('11011001')  BitMaskRealWorld=Stored Integer
  Bitwise_And2 : simulink/Logic and Bit Operations/Bitwise Operator  logicop=AND  UseBitMask=off  BitMask=bin2dec('11011001')  BitMaskRealWorld=Stored Integer
  Bitwise_And3 : simulink/Logic and Bit Operations/Bitwise Operator  logicop=AND  UseBitMask=off  BitMask=bin2dec('11011001')  BitMaskRealWorld=Stored Integer
  Scope : Scope  NumInputPorts=3
  Scope1 : Scope  NumInputPorts=2
  Scope2 : Scope  NumInputPorts=2
  Scope3 : Scope  NumInputPorts=2
  cmp_1 : UnitTest_Lib/RoughlyEqual  slope=1
  cmp_2 : UnitTest_Lib/RoughlyEqual  slope=0.1
  cmp_3 : UnitTest_Lib/RoughlyEqual  slope=1
  result_tws : ToWorkspace  VariableName=spec_result_002
  tws_1 : ToWorkspace  VariableName=spec_req_002_001
  tws_2 : ToWorkspace  VariableName=spec_req_002_002
  tws_3 : ToWorkspace  VariableName=spec_req_002_003
  result : Outport
  wires:
  sig_Req_Bus/1 -> BS_Req/1
  sig_Result_Bus/1 -> BS_Result/1
  AndN/1 -> result/1, result_tws/1
  BS_Req/1 -> cmp_1/1, Scope1/1  "<testSig_EngPrt_trqLimMech>"
  BS_Result/1 -> cmp_1/2, Scope1/2  "<EngPrt_trqLimMech>"
  cmp_1/1 -> Bitwise_And1/1
  Bitwise_And1/1 -> AndN/1, Scope/1, tws_1/1
  BS_Req/2 -> cmp_2/1, Scope2/1  "<testSig_EngPrt_trqUnLim>"
  BS_Result/2 -> cmp_2/2, Scope2/2  "<EngPrt_trqUnLim>"
  cmp_2/1 -> Bitwise_And2/1
  Bitwise_And2/1 -> AndN/2, Scope/2, tws_2/1
  BS_Req/3 -> cmp_3/1, Scope3/1  "<testSig_EngPrt_trqNLim>"
  BS_Result/3 -> cmp_3/2, Scope3/2  "<EngPrt_trqNLim>"
  cmp_3/1 -> Bitwise_And3/1
  Bitwise_And3/1 -> AndN/3, Scope/3, tws_3/1

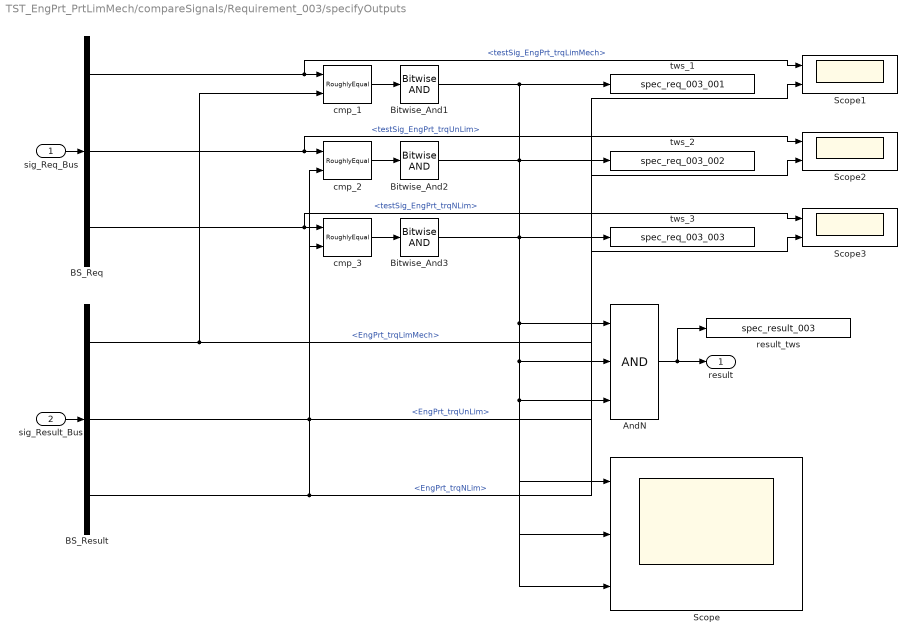
== system TST_EngPrt_PrtLimMech/compareSignals/Requirement_003/specifyOutputs ==
  sig_Req_Bus : Inport
  sig_Result_Bus : Inport  Port=2
  AndN : Logic  Inputs=3
  BS_Req : BusSelector  OutputSignals=testSig_EngPrt_trqLimMech,testSig_EngPrt_trqUnLim,testSig_EngPrt_trqNLim
  BS_Result : BusSelector  OutputSignals=EngPrt_trqLimMech,EngPrt_trqUnLim,EngPrt_trqNLim
  Bitwise_And1 : simulink/Logic and Bit Operations/Bitwise Operator  logicop=AND  UseBitMask=off  BitMask=bin2dec('11011001')  BitMaskRealWorld=Stored Integer
  Bitwise_And2 : simulink/Logic and Bit Operations/Bitwise Operator  logicop=AND  UseBitMask=off  BitMask=bin2dec('11011001')  BitMaskRealWorld=Stored Integer
  Bitwise_And3 : simulink/Logic and Bit Operations/Bitwise Operator  logicop=AND  UseBitMask=off  BitMask=bin2dec('11011001')  BitMaskRealWorld=Stored Integer
  Scope : Scope  NumInputPorts=3
  Scope1 : Scope  NumInputPorts=2
  Scope2 : Scope  NumInputPorts=2
  Scope3 : Scope  NumInputPorts=2
  cmp_1 : UnitTest_Lib/RoughlyEqual  slope=1
  cmp_2 : UnitTest_Lib/RoughlyEqual  slope=0.1
  cmp_3 : UnitTest_Lib/RoughlyEqual  slope=1
  result_tws : ToWorkspace  VariableName=spec_result_003
  tws_1 : ToWorkspace  VariableName=spec_req_003_001
  tws_2 : ToWorkspace  VariableName=spec_req_003_002
  tws_3 : ToWorkspace  VariableName=spec_req_003_003
  result : Outport
  wires:
  sig_Req_Bus/1 -> BS_Req/1
  sig_Result_Bus/1 -> BS_Result/1
  AndN/1 -> result/1, result_tws/1
  BS_Req/1 -> cmp_1/1, Scope1/1  "<testSig_EngPrt_trqLimMech>"
  BS_Result/1 -> cmp_1/2, Scope1/2  "<EngPrt_trqLimMech>"
  cmp_1/1 -> Bitwise_And1/1
  Bitwise_And1/1 -> AndN/1, Scope/1, tws_1/1
  BS_Req/2 -> cmp_2/1, Scope2/1  "<testSig_EngPrt_trqUnLim>"
  BS_Result/2 -> cmp_2/2, Scope2/2  "<EngPrt_trqUnLim>"
  cmp_2/1 -> Bitwise_And2/1
  Bitwise_And2/1 -> AndN/2, Scope/2, tws_2/1
  BS_Req/3 -> cmp_3/1, Scope3/1  "<testSig_EngPrt_trqNLim>"
  BS_Result/3 -> cmp_3/2, Scope3/2  "<EngPrt_trqNLim>"
  cmp_3/1 -> Bitwise_And3/1
  Bitwise_And3/1 -> AndN/3, Scope/3, tws_3/1

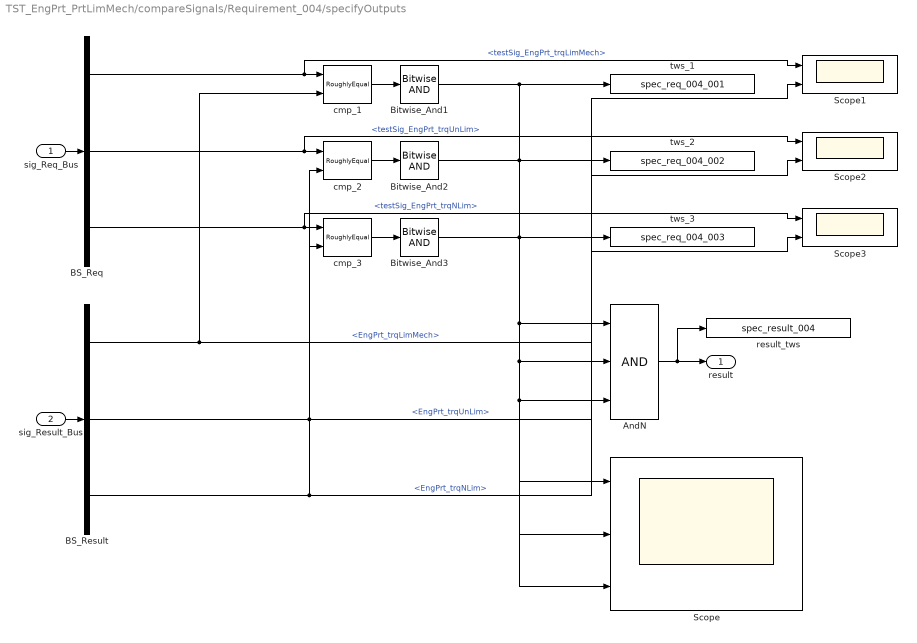
== system TST_EngPrt_PrtLimMech/compareSignals/Requirement_004/specifyOutputs ==
  sig_Req_Bus : Inport
  sig_Result_Bus : Inport  Port=2
  AndN : Logic  Inputs=3
  BS_Req : BusSelector  OutputSignals=testSig_EngPrt_trqLimMech,testSig_EngPrt_trqUnLim,testSig_EngPrt_trqNLim
  BS_Result : BusSelector  OutputSignals=EngPrt_trqLimMech,EngPrt_trqUnLim,EngPrt_trqNLim
  Bitwise_And1 : simulink/Logic and Bit Operations/Bitwise Operator  logicop=AND  UseBitMask=off  BitMask=bin2dec('11011001')  BitMaskRealWorld=Stored Integer
  Bitwise_And2 : simulink/Logic and Bit Operations/Bitwise Operator  logicop=AND  UseBitMask=off  BitMask=bin2dec('11011001')  BitMaskRealWorld=Stored Integer
  Bitwise_And3 : simulink/Logic and Bit Operations/Bitwise Operator  logicop=AND  UseBitMask=off  BitMask=bin2dec('11011001')  BitMaskRealWorld=Stored Integer
  Scope : Scope  NumInputPorts=3
  Scope1 : Scope  NumInputPorts=2
  Scope2 : Scope  NumInputPorts=2
  Scope3 : Scope  NumInputPorts=2
  cmp_1 : UnitTest_Lib/RoughlyEqual  slope=1
  cmp_2 : UnitTest_Lib/RoughlyEqual  slope=0.1
  cmp_3 : UnitTest_Lib/RoughlyEqual  slope=1
  result_tws : ToWorkspace  VariableName=spec_result_004
  tws_1 : ToWorkspace  VariableName=spec_req_004_001
  tws_2 : ToWorkspace  VariableName=spec_req_004_002
  tws_3 : ToWorkspace  VariableName=spec_req_004_003
  result : Outport
  wires:
  sig_Req_Bus/1 -> BS_Req/1
  sig_Result_Bus/1 -> BS_Result/1
  AndN/1 -> result/1, result_tws/1
  BS_Req/1 -> cmp_1/1, Scope1/1  "<testSig_EngPrt_trqLimMech>"
  BS_Result/1 -> cmp_1/2, Scope1/2  "<EngPrt_trqLimMech>"
  cmp_1/1 -> Bitwise_And1/1
  Bitwise_And1/1 -> AndN/1, Scope/1, tws_1/1
  BS_Req/2 -> cmp_2/1, Scope2/1  "<testSig_EngPrt_trqUnLim>"
  BS_Result/2 -> cmp_2/2, Scope2/2  "<EngPrt_trqUnLim>"
  cmp_2/1 -> Bitwise_And2/1
  Bitwise_And2/1 -> AndN/2, Scope/2, tws_2/1
  BS_Req/3 -> cmp_3/1, Scope3/1  "<testSig_EngPrt_trqNLim>"
  BS_Result/3 -> cmp_3/2, Scope3/2  "<EngPrt_trqNLim>"
  cmp_3/1 -> Bitwise_And3/1
  Bitwise_And3/1 -> AndN/3, Scope/3, tws_3/1
